simulink model "ActiveSupensionTsModel"  (R2014a)
settings: Solver=ode4  StartTime=0.0  StopTime=5  FixedStep=0.001  RelTol=1e-3
settings Model: Creator=MLRida  LastModifiedBy=MLRida

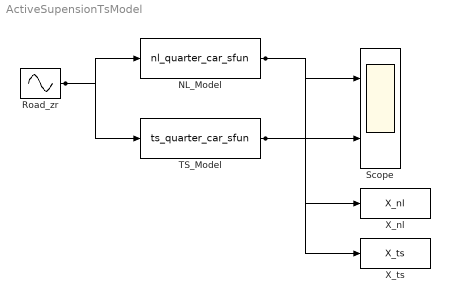
== system ActiveSupensionTsModel ==
  NL_Model : S-Function  FunctionName=nl_quarter_car_sfun  EnableBusSupport=off
  Road_zr : Sin  Amplitude=0.05  Frequency=12.566  SampleTime=0
  Scope : Scope  NumInputPorts=2
  TS_Model : S-Function  FunctionName=ts_quarter_car_sfun  EnableBusSupport=off
  X_nl : ToWorkspace  VariableName=X_nl  SampleTime=-1
  X_ts : ToWorkspace  VariableName=X_ts  SampleTime=-1
  wires:
  Road_zr/1 -> NL_Model/1, TS_Model/1
  NL_Model/1 -> Scope/1, X_nl/1
  TS_Model/1 -> Scope/2, X_ts/1
